simulink model "Test8"  (R2021b)
settings: Solver=FixedStepAuto  StartTime=0.0  StopTime=Inf  RelTol=1e-3  EnableMultiTasking=on
undefined symbols (not defined in the file): magnitude
libraries: arduinolib x8
settings Model: ExtModeTrigDuration=2  Creator=diego  LastModifiedBy=diego
settings OptimizationCC: EnhancedBackFolding=on  PassReuseOutputArgsAs=Individual arguments  ZeroExternalMemoryAtStartup=off  ZeroInternalMemoryAtStartup=off  MaxStackSize=64  OptimizeBlockOrder=speed  DifferentSizesBufferReuse=on  EfficientTunableParamExpr=on
settings DebuggingCC: ParameterTunabilityLossMsg=error
settings HardwareCC: ProdBitPerInt=16  ProdBitPerPointer=16  ProdBitPerSizeT=16  ProdBitPerPtrDiffT=16  ProdLargestAtomicFloat=None  ProdWordSize=8  ProdHWDeviceType=Atmel->AVR
settings SFSimCC: MATLABDynamicMemAlloc=off
settings RTWCC: Description=Embedded Coder  SystemTargetFile=ert.tlc  HardwareBoard=Arduino Uno  TemplateMakefile=ert_default_tmf  Toolchain=Arduino AVR  BuildConfiguration=Faster Runs
settings CodeAppCC: ForceParamTrailComments=on  IgnoreCustomStorageClasses=off  OperatorAnnotations=on  SimulinkDataObjDesc=on  SFDataObjDesc=on  InsertBlockDesc=on
settings ERTTargetCC: SupportContinuousTime=on  SupportVariableSizeSignals=on  ExtModeTransport=3  ExtModeStaticAlloc=on  ExtModeStaticAllocSize=250  ExtModeMexFile=ext_xcp  ExtModeIntrfLevel=Level2 - Open

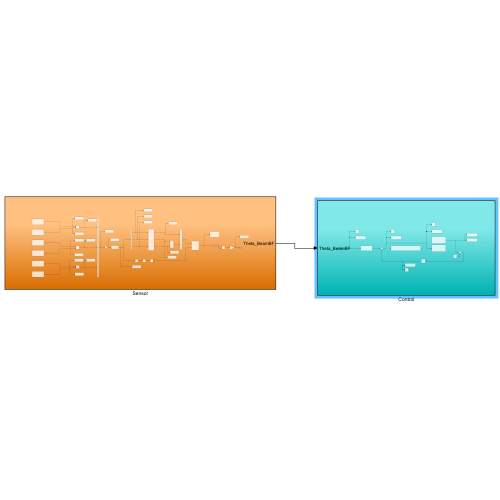
[thumbnail: Simulink's stored preview of the top-level diagram]
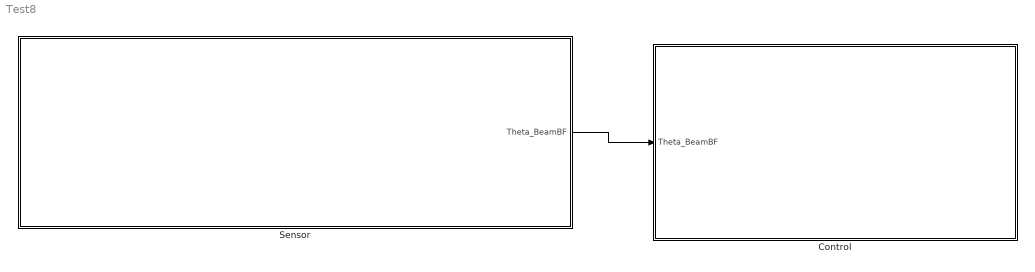
== system Test8 ==
  Control : Subsystem
  Sensor : Subsystem
  wires:
  Sensor/1(Theta_BeamBF) -> Control/1(Theta_BeamBF)

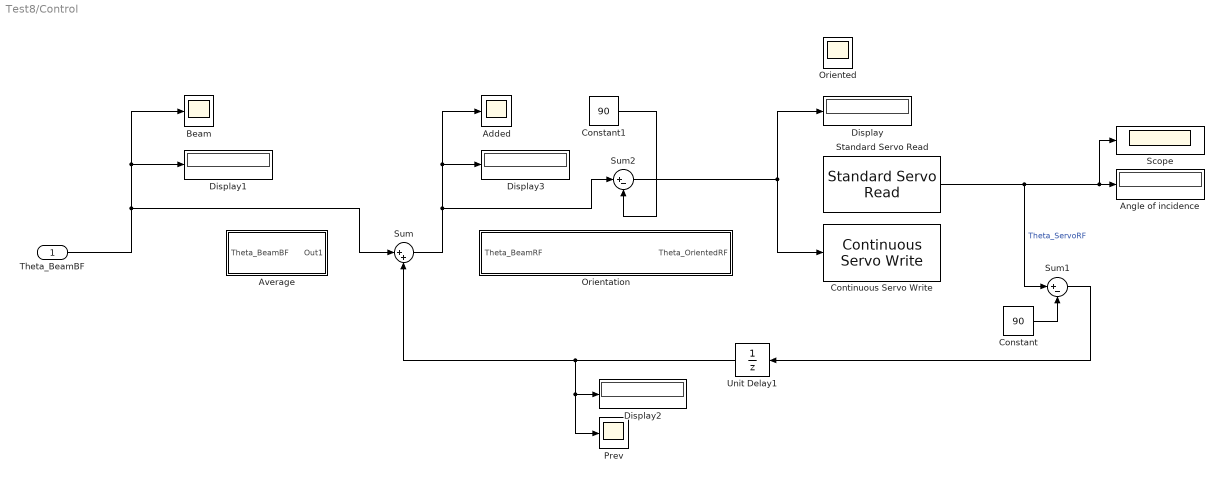
== system Test8/Control ==
  Theta_BeamBF : Inport
  Added : Scope
  Angle of incidence : Display
  Average : Subsystem
  Beam : Scope
  Constant : Constant  Value=90
  Constant1 : Constant  Value=90
  Continuous Servo Write : arduinolib/Continuous Servo Write  pinNumber=9  ServoIndex=0  blockPlatform=ARDUINO
      settings: SourceProductBaseCode=ARDUINO
  Display{,1..3} (4 alike) : Display
  Orientation : Subsystem
  Oriented : Scope
  Prev : Scope
  Scope : Scope
  Standard Servo Read : arduinolib/Standard Servo Read  pinNumber=9  SampleTime=0.1  ServoIndex=0  blockPlatform=ARDUINO
      settings: SourceProductBaseCode=ARDUINO
  Sum : Sum  Inputs=|++
  Sum1 : Sum  Inputs=|+-
  Sum2 : Sum  Inputs=|+-
  Unit Delay1 : UnitDelay  SampleTime=-1  HasFrameUpgradeWarning=on
  wires:
  Sum/1 -> Sum2/1, Display3/1, Added/1
  Standard Servo Read/1 -> Scope/1, Angle of incidence/1, Sum1/1  "Theta_ServoRF"
  Unit Delay1/1 -> Prev/1, Display2/1, Sum/2
  Theta_BeamBF/1 -> Sum/1, Beam/1, Display1/1
  Sum1/1 -> Unit Delay1/1
  Constant/1 -> Sum1/2
  Sum2/1 -> Continuous Servo Write/1, Display/1
  Constant1/1 -> Sum2/2

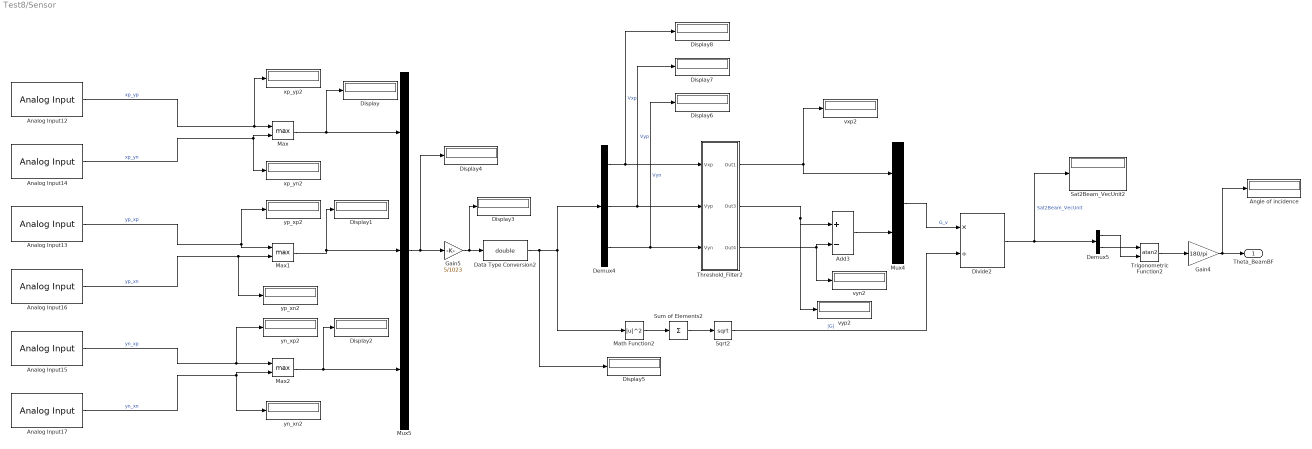
== system Test8/Sensor ==
  Add3 : Sum  Inputs=+|-
  Analog Input12 : arduinolib/Analog Input  pinNumber=3  ReadResultsOnly=off  ConversionTriggerSource=Software  ExternalTriggerType=uint32( 0 )  OutputDataType=uint16  EnableConversionCompleteNotify=off  EnableOuputStatus=off  SampleTime=-1  blockPlatform=arduino
  Analog Input13 : arduinolib/Analog Input  pinNumber=4  ReadResultsOnly=off  ConversionTriggerSource=Software  ExternalTriggerType=uint32( 0 )  OutputDataType=uint16  EnableConversionCompleteNotify=off  EnableOuputStatus=off  SampleTime=-1  blockPlatform=arduino
  Analog Input14 : arduinolib/Analog Input  pinNumber=2  ReadResultsOnly=off  ConversionTriggerSource=Software  ExternalTriggerType=uint32( 0 )  OutputDataType=uint16  EnableConversionCompleteNotify=off  EnableOuputStatus=off  SampleTime=-1  blockPlatform=arduino
  Analog Input15 : arduinolib/Analog Input  pinNumber=1  ReadResultsOnly=off  ConversionTriggerSource=Software  ExternalTriggerType=uint32( 0 )  OutputDataType=uint16  EnableConversionCompleteNotify=off  EnableOuputStatus=off  SampleTime=-1  blockPlatform=arduino
  Analog Input16 : arduinolib/Analog Input  pinNumber=5  ReadResultsOnly=off  ConversionTriggerSource=Software  ExternalTriggerType=uint32( 0 )  OutputDataType=uint16  EnableConversionCompleteNotify=off  EnableOuputStatus=off  SampleTime=-1  blockPlatform=arduino
  Analog Input17 : arduinolib/Analog Input  pinNumber=0  ReadResultsOnly=off  ConversionTriggerSource=Software  ExternalTriggerType=uint32( 0 )  OutputDataType=uint16  EnableConversionCompleteNotify=off  EnableOuputStatus=off  SampleTime=-1  blockPlatform=arduino
  Angle of incidence : Display
  Data Type Conversion2 : DataTypeConversion  OutDataTypeStr=double
  Demux4 : Demux  Outputs=3
  Demux5 : Demux  Outputs=2
  Display{,1..8} (9 alike) : Display
  Divide2 : Product  Inputs=*/
  Gain4 : Gain  Gain=180/pi
  Gain5 : Gain  Gain=5/1023
  Math Function2 : Math  Operator=magnitude^2  OutputSignalType=real  SaturateOnIntegerOverflow=on
  Max : MinMax  Function=max  Inputs=2
  Max1 : MinMax  Function=max  Inputs=2
  Max2 : MinMax  Function=max  Inputs=2
  Mux4 : Mux  Inputs=2
  Mux5 : Mux  Inputs=3
  Sat2Beam_VecUnit2 : Display
  Sqrt2 : Sqrt  SaturateOnIntegerOverflow=on
  Sum of Elements2 : Sum  Inputs=+
  Threshold_Filter2 : Subsystem
  Trigonometric Function2 : Trigonometry  Operator=atan2
  vxp2 : Display
  vyn2 : Display
  vyp2 : Display
  xp_yn2 : Display
  xp_yp2 : Display
  yn_xn2 : Display
  yn_xp2 : Display
  yp_xn2 : Display
  yp_xp2 : Display
  Theta_BeamBF : Outport
  wires:
  Data Type Conversion2/1 -> Display5/1, Math Function2/1, Demux4/1
  Demux4/2 -> Display7/1, Threshold_Filter2/2(Vyp)  "Vyp"
  Trigonometric Function2/1 -> Gain4/1
  Analog Input12/1 -> Max/1, xp_yp2/1  "xp_yp"
  Threshold_Filter2/1(Out1) -> Mux4/1, vxp2/1
  Mux5/1 -> Display4/1, Gain5/1
  Divide2/1 -> Demux5/1, Sat2Beam_VecUnit2/1  "Sat2Beam_VecUnit"
  Demux4/3 -> Display6/1, Threshold_Filter2/3(Vyn)  "Vyn"
  Gain5/1 -> Display3/1, Data Type Conversion2/1
  Analog Input14/1 -> xp_yn2/1, Max/2  "xp_yn"
  Sqrt2/1 -> Divide2/2  "|G|"
  Demux5/1 -> Trigonometric Function2/2
  Demux4/1 -> Display8/1, Threshold_Filter2/1(Vxp)  "Vxp"
  Threshold_Filter2/3(Out4) -> vyn2/1, Add3/2
  Add3/1 -> Mux4/2
  Analog Input15/1 -> Max2/1, yn_xp2/1  "yn_xp"
  Analog Input13/1 -> Max1/1, yp_xp2/1  "yp_xp"
  Threshold_Filter2/2(Out3) -> vyp2/1, Add3/1
  Mux4/1 -> Divide2/1  "G_v"
  Demux5/2 -> Trigonometric Function2/1
  Sum of Elements2/1 -> Sqrt2/1
  Math Function2/1 -> Sum of Elements2/1
  Analog Input17/1 -> Max2/2, yn_xn2/1  "yn_xn"
  Analog Input16/1 -> Max1/2, yp_xn2/1  "yp_xn"
  Max1/1 -> Display1/1, Mux5/2
  Max/1 -> Display/1, Mux5/1
  Max2/1 -> Display2/1, Mux5/3
  Gain4/1 -> Angle of incidence/1, Theta_BeamBF/1

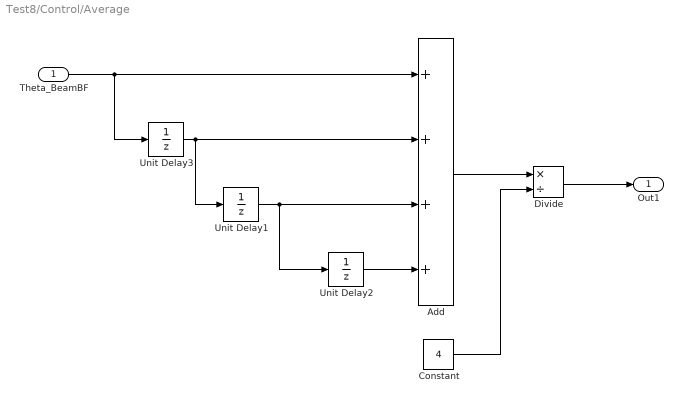
== system Test8/Control/Average ==
  Theta_BeamBF : Inport
  Add : Sum  Inputs=++++
  Constant : Constant  Value=4
  Divide : Product  Inputs=*/
  Unit Delay1 : UnitDelay  SampleTime=-1  HasFrameUpgradeWarning=on
  Unit Delay2 : UnitDelay  SampleTime=-1  HasFrameUpgradeWarning=on
  Unit Delay3 : UnitDelay  SampleTime=-1  HasFrameUpgradeWarning=on
  Out1 : Outport
  wires:
  Unit Delay3/1 -> Unit Delay1/1, Add/2
  Add/1 -> Divide/1
  Constant/1 -> Divide/2
  Theta_BeamBF/1 -> Add/1, Unit Delay3/1
  Unit Delay1/1 -> Unit Delay2/1, Add/3
  Unit Delay2/1 -> Add/4
  Divide/1 -> Out1/1

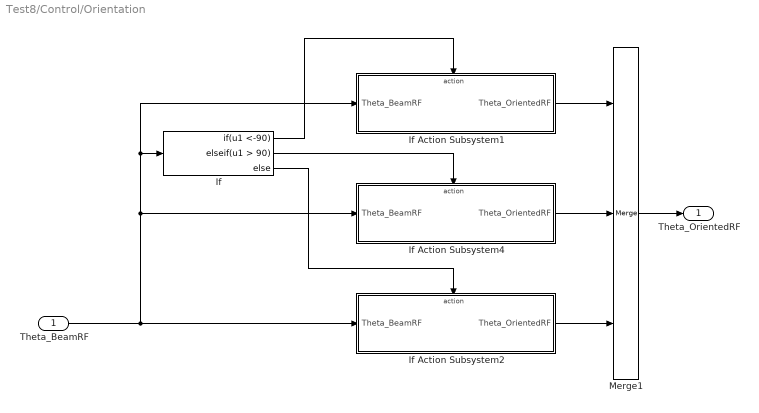
== system Test8/Control/Orientation ==
  Theta_BeamRF : Inport
  If : If  IfExpression=u1 <-90  ElseIfExpressions=u1 > 90
  If Action Subsystem1 : Subsystem  TreatAsAtomicUnit=on
  If Action Subsystem2 : Subsystem  TreatAsAtomicUnit=on
  If Action Subsystem4 : Subsystem  TreatAsAtomicUnit=on
  Merge1 : Merge  Inputs=3
  Theta_OrientedRF : Outport
  wires:
  If Action Subsystem1/1(Theta_OrientedRF) -> Merge1/1
  Merge1/1 -> Theta_OrientedRF/1
  If/1 -> If Action Subsystem1/Action
  Theta_BeamRF/1 -> If Action Subsystem2/1(Theta_BeamRF), If Action Subsystem4/1(Theta_BeamRF), If Action Subsystem1/1(Theta_BeamRF), If/1
  If/2 -> If Action Subsystem4/Action
  If/3 -> If Action Subsystem2/Action
  If Action Subsystem4/1(Theta_OrientedRF) -> Merge1/2
  If Action Subsystem2/1(Theta_OrientedRF) -> Merge1/3

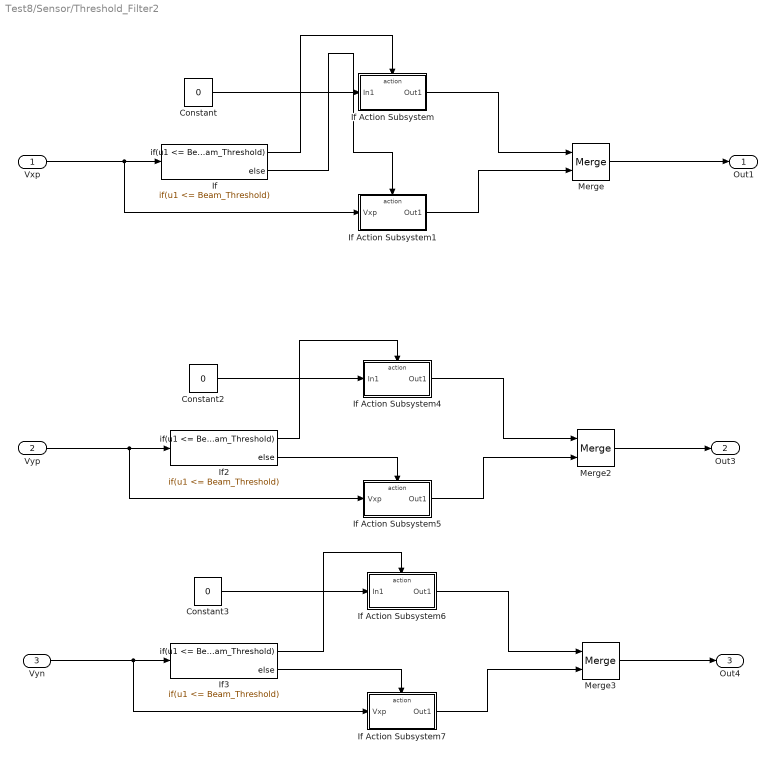
== system Test8/Sensor/Threshold_Filter2 ==
  Vxp : Inport
  Vyp : Inport  Port=2
  Vyn : Inport  Port=3
  Constant : Constant  Value=0
  Constant2 : Constant  Value=0
  Constant3 : Constant  Value=0
  If : If  IfExpression=u1 <= Beam_Threshold
  If Action Subsystem : Subsystem  TreatAsAtomicUnit=on
  If Action Subsystem1 : Subsystem  TreatAsAtomicUnit=on
  If Action Subsystem4 : Subsystem  TreatAsAtomicUnit=on
  If Action Subsystem5 : Subsystem  TreatAsAtomicUnit=on
  If Action Subsystem6 : Subsystem  TreatAsAtomicUnit=on
  If Action Subsystem7 : Subsystem  TreatAsAtomicUnit=on
  If2 : If  IfExpression=u1 <= Beam_Threshold
  If3 : If  IfExpression=u1 <= Beam_Threshold
  Merge : Merge
  Merge2 : Merge
  Merge3 : Merge
  Out1 : Outport
  Out3 : Outport  Port=2
  Out4 : Outport  Port=3
  wires:
  Vxp/1 -> If Action Subsystem1/1(Vxp), If/1
  If/1 -> If Action Subsystem/Action
  If Action Subsystem/1(Out1) -> Merge/1
  If/2 -> If Action Subsystem1/Action
  If Action Subsystem1/1(Out1) -> Merge/2
  Merge/1 -> Out1/1
  Constant/1 -> If Action Subsystem/1(In1)
  Vyp/1 -> If2/1, If Action Subsystem5/1(Vxp)
  If2/2 -> If Action Subsystem5/Action
  If2/1 -> If Action Subsystem4/Action
  If Action Subsystem4/1(Out1) -> Merge2/1
  If Action Subsystem5/1(Out1) -> Merge2/2
  Constant2/1 -> If Action Subsystem4/1(In1)
  Merge2/1 -> Out3/1
  Vyn/1 -> If3/1, If Action Subsystem7/1(Vxp)
  Merge3/1 -> Out4/1
  If Action Subsystem7/1(Out1) -> Merge3/2
  If3/2 -> If Action Subsystem7/Action
  If Action Subsystem6/1(Out1) -> Merge3/1
  Constant3/1 -> If Action Subsystem6/1(In1)
  If3/1 -> If Action Subsystem6/Action

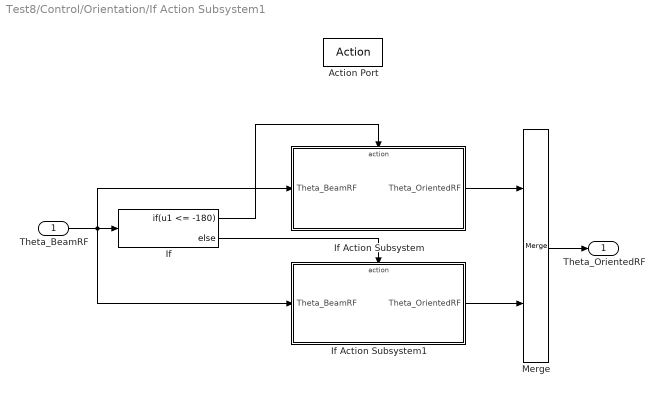
== system Test8/Control/Orientation/If Action Subsystem1 ==
  Theta_BeamRF : Inport
  Action Port : ActionPort  ActionPortLabel=if(u1 <-90)
  If : If  IfExpression=u1 <= -180
  If Action Subsystem : Subsystem  TreatAsAtomicUnit=on
  If Action Subsystem1 : Subsystem  TreatAsAtomicUnit=on
  Merge : Merge
  Theta_OrientedRF : Outport
  wires:
  Theta_BeamRF/1 -> If Action Subsystem/1(Theta_BeamRF), If Action Subsystem1/1(Theta_BeamRF), If/1
  Merge/1 -> Theta_OrientedRF/1
  If Action Subsystem/1(Theta_OrientedRF) -> Merge/1
  If Action Subsystem1/1(Theta_OrientedRF) -> Merge/2
  If/1 -> If Action Subsystem/Action
  If/2 -> If Action Subsystem1/Action

== system Test8/Control/Orientation/If Action Subsystem2 ==
  Theta_BeamRF : Inport
  Action Port : ActionPort  ActionPortLabel=else
  Theta_OrientedRF : Outport
  wires:
  Theta_BeamRF/1 -> Theta_OrientedRF/1

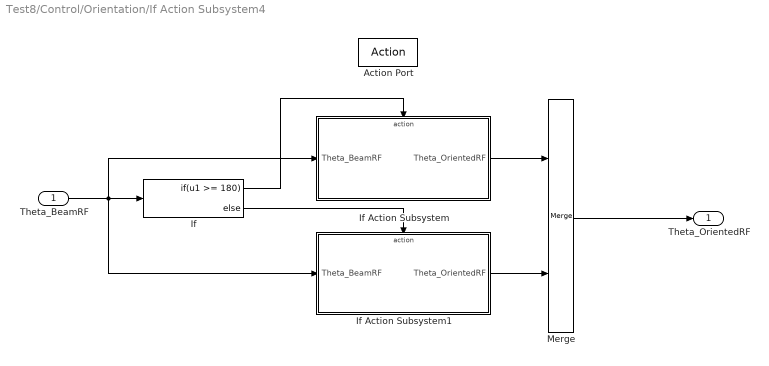
== system Test8/Control/Orientation/If Action Subsystem4 ==
  Theta_BeamRF : Inport
  Action Port : ActionPort  ActionPortLabel=elseif(u1 > 90)
  If : If  IfExpression=u1 >= 180
  If Action Subsystem : Subsystem  TreatAsAtomicUnit=on
  If Action Subsystem1 : Subsystem  TreatAsAtomicUnit=on
  Merge : Merge
  Theta_OrientedRF : Outport
  wires:
  Merge/1 -> Theta_OrientedRF/1
  If Action Subsystem/1(Theta_OrientedRF) -> Merge/1
  If Action Subsystem1/1(Theta_OrientedRF) -> Merge/2
  If/1 -> If Action Subsystem/Action
  If/2 -> If Action Subsystem1/Action
  Theta_BeamRF/1 -> If/1, If Action Subsystem1/1(Theta_BeamRF), If Action Subsystem/1(Theta_BeamRF)

== system Test8/Sensor/Threshold_Filter2/If Action Subsystem ==
  In1 : Inport
  Action Port : ActionPort  ActionPortLabel=if(u1 <= Beam_Threshold)
  Out1 : Outport
  wires:
  In1/1 -> Out1/1

== system Test8/Sensor/Threshold_Filter2/If Action Subsystem1 ==
  Vxp : Inport
  Action Port : ActionPort  ActionPortLabel=else
  Out1 : Outport
  wires:
  Vxp/1 -> Out1/1

== system Test8/Sensor/Threshold_Filter2/If Action Subsystem4 ==
  In1 : Inport
  Action Port : ActionPort  ActionPortLabel=if(u1 <= Beam_Threshold)
  Out1 : Outport
  wires:
  In1/1 -> Out1/1

== system Test8/Sensor/Threshold_Filter2/If Action Subsystem5 ==
  Vxp : Inport
  Action Port : ActionPort  ActionPortLabel=else
  Out1 : Outport
  wires:
  Vxp/1 -> Out1/1

== system Test8/Sensor/Threshold_Filter2/If Action Subsystem6 ==
  In1 : Inport
  Action Port : ActionPort  ActionPortLabel=if(u1 <= Beam_Threshold)
  Out1 : Outport
  wires:
  In1/1 -> Out1/1

== system Test8/Sensor/Threshold_Filter2/If Action Subsystem7 ==
  Vxp : Inport
  Action Port : ActionPort  ActionPortLabel=else
  Out1 : Outport
  wires:
  Vxp/1 -> Out1/1

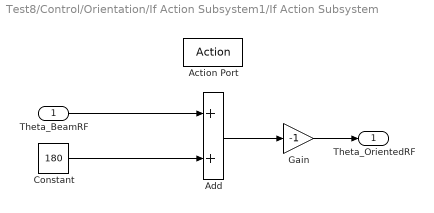
== system Test8/Control/Orientation/If Action Subsystem1/If Action Subsystem ==
  Theta_BeamRF : Inport
  Action Port : ActionPort  ActionPortLabel=if(u1 <= -180)
  Add : Sum
  Constant : Constant  Value=180
  Gain : Gain  Gain=-1
  Theta_OrientedRF : Outport
  wires:
  Constant/1 -> Add/2
  Gain/1 -> Theta_OrientedRF/1
  Add/1 -> Gain/1
  Theta_BeamRF/1 -> Add/1

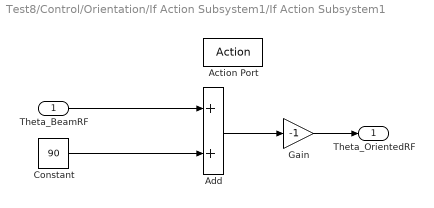
== system Test8/Control/Orientation/If Action Subsystem1/If Action Subsystem1 ==
  Theta_BeamRF : Inport
  Action Port : ActionPort  ActionPortLabel=else
  Add : Sum
  Constant : Constant  Value=90
  Gain : Gain  Gain=-1
  Theta_OrientedRF : Outport
  wires:
  Constant/1 -> Add/2
  Add/1 -> Gain/1
  Gain/1 -> Theta_OrientedRF/1
  Theta_BeamRF/1 -> Add/1

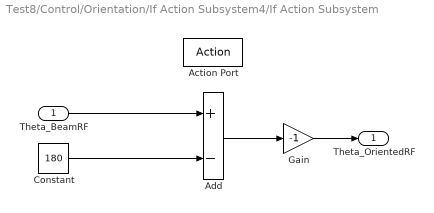
== system Test8/Control/Orientation/If Action Subsystem4/If Action Subsystem ==
  Theta_BeamRF : Inport
  Action Port : ActionPort  ActionPortLabel=if(u1 >= 180)
  Add : Sum  Inputs=+-
  Constant : Constant  Value=180
  Gain : Gain  Gain=-1
  Theta_OrientedRF : Outport
  wires:
  Constant/1 -> Add/2
  Gain/1 -> Theta_OrientedRF/1
  Add/1 -> Gain/1
  Theta_BeamRF/1 -> Add/1

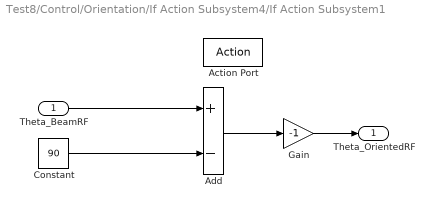
== system Test8/Control/Orientation/If Action Subsystem4/If Action Subsystem1 ==
  Theta_BeamRF : Inport
  Action Port : ActionPort  ActionPortLabel=else
  Add : Sum  Inputs=+-
  Constant : Constant  Value=90
  Gain : Gain  Gain=-1
  Theta_OrientedRF : Outport
  wires:
  Constant/1 -> Add/2
  Add/1 -> Gain/1
  Gain/1 -> Theta_OrientedRF/1
  Theta_BeamRF/1 -> Add/1
